simulink model "TST_SfVariableInputTest"  (Simulink 7.4)
settings: Solver=FixedStepDiscrete  StartTime=0.0  StopTime=10.0  FixedStep=0.02  RelTol=1e-3
settings Model: Creator=kharthforeign  LastModifiedBy=kharthforeign  BufferReuse=off
settings DataIOCC: SaveOutput=off  SignalLogging=off  SaveTime=off
settings OptimizationCC: BlockReduction=off  ConditionallyExecuteInputs=off  OptimizeBlockIOStorage=off  BufferReuse=off  ExpressionFolding=off  LocalBlockOutputs=off  InitFltsAndDblsToZero=on
settings RTWCC: GenCodeOnly=on

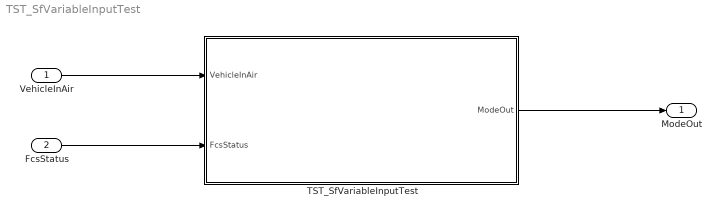
== system TST_SfVariableInputTest ==
  VehicleInAir : Inport  PortDimensions=1  DataType=boolean  OutDataType=fixdt(1, 16)  OutScaling=2^0  OutDataTypeStr=boolean
  FcsStatus : Inport  Port=2  UseBusObject=on  OutDataType=fixdt(1, 16)  OutScaling=2^0
      settings: BusObject=FCS_FlightControlSystem_Status
  TST_SfVariableInputTest : Subsystem  TreatAsAtomicUnit=on
  ModeOut : Outport  PortDimensions=1  DataType=int32  OutDataType=Enum: GBL_Definitions_EjectionCmd  OutDataTypeStr=int32
  wires:
  VehicleInAir/1 -> TST_SfVariableInputTest/1(VehicleInAir)
  FcsStatus/1 -> TST_SfVariableInputTest/2(FcsStatus)
  TST_SfVariableInputTest/1(ModeOut) -> ModeOut/1

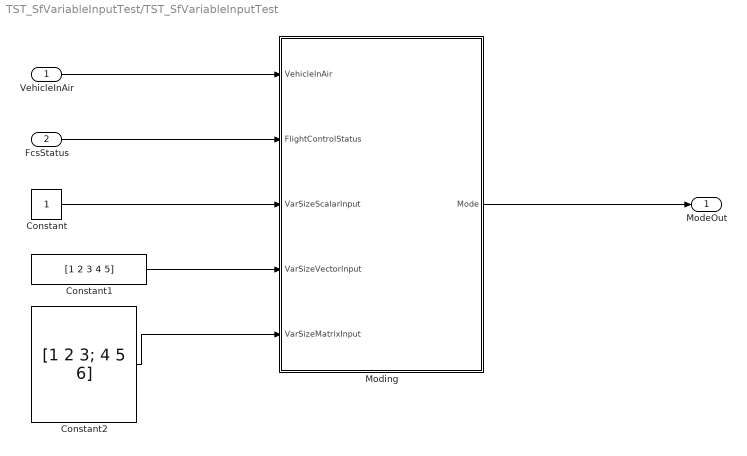
== system TST_SfVariableInputTest/TST_SfVariableInputTest ==
  VehicleInAir : Inport  PortDimensions=1  DataType=boolean  OutDataType=fixdt(1, 16)  OutScaling=2^0  OutDataTypeStr=boolean
  FcsStatus : Inport  Port=2  UseBusObject=on  OutDataType=fixdt(1, 16)  OutScaling=2^0
      settings: BusObject=FCS_FlightControlSystem_Status
  Constant : Constant  OutDataType=fixdt(1, 16)  OutScaling=2^0
  Constant1 : Constant  Value=[1 2 3 4 5]  OutDataType=fixdt(1, 16)  OutScaling=2^0
  Constant2 : Constant  Value=[1 2 3; 4 5 6]  VectorParams1D=off  OutDataType=fixdt(1, 16)  OutScaling=2^0
  Moding : Stateflow chart  TreatAsAtomicUnit=on
  ModeOut : Outport  PortDimensions=1  DataType=int32  OutDataType=Enum: GBL_Definitions_EjectionCmd  OutDataTypeStr=int32
  wires:
  FcsStatus/1 -> Moding/2(FlightControlStatus)
  VehicleInAir/1 -> Moding/1(VehicleInAir)
  Moding/1(Mode) -> ModeOut/1
  Constant/1 -> Moding/3(VarSizeScalarInput)
  Constant1/1 -> Moding/4(VarSizeVectorInput)
  Constant2/1 -> Moding/5(VarSizeMatrixInput)

== stateflow chart TST_SfVariableInputTest/Moding ==
  state TopStateA
    during:
    Mode = int32(111);
    state Launch
      entry:
      Mode = int32(VarSizeVectorInput[2]);
    state Off
      entry:
      Mode = int32(1);
    (default) -> Off
    Off -> Launch : [(FlightControlStatus.PressureAltitude_Ft < 500.0) && (~VehicleInAir)]
  (default) -> TopStateA
  data: VehicleInAir input boolean; Mode output int32; FlightControlStatus input FCS_FlightControlSystem_Status; VarSizeScalarInput input double; VarSizeVectorInput input double; VarSizeMatrixInput input double
